simulink subsystem "KF_prediction"  (R2021a)
settings: Solver=VariableStepAuto  StartTime=0.0  StopTime=10.0  RelTol=1e-3
undefined symbols (not defined in the file): gyro_bias_init, gyro_std, magnitude
libraries: dspmtrx3 x5
settings Model: Creator=Laura  LastModifiedBy=Laura

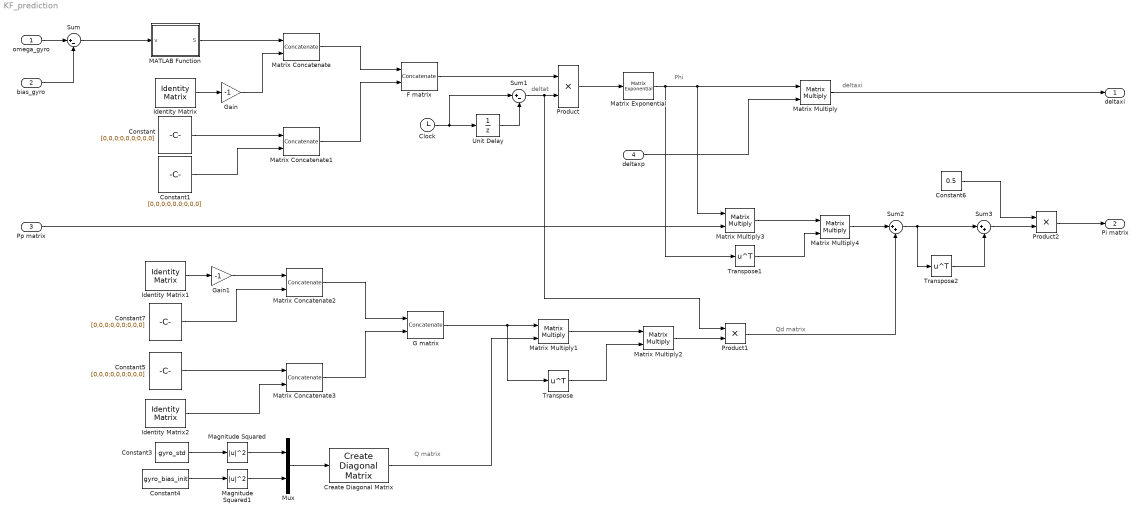
== system KF_prediction ==
  note: Qd matrix
  note: Q matrix
  note: Phi
  note: deltaxi
  note: deltat
  omega_gyro : Inport
  bias_gyro : Inport  Port=2
  Pp matrix : Inport  Port=3
  deltaxp : Inport  Port=4
  Clock : Clock
  Constant{,1,5,7} (4 alike) : Constant  Value=[0,0,0;0,0,0;0,0,0]
  Constant3 : Constant  Value=gyro_std
  Constant4 : Constant  Value=gyro_bias_init
  Constant6 : Constant  Value=0.5
  Create Diagonal Matrix : dspmtrx3/Create Diagonal Matrix
      settings: SourceProductBaseCode=DS
  F matrix : Concatenate  Mode=Multidimensional array
  G matrix : Concatenate  Mode=Multidimensional array
  Gain : Gain  Gain=-1
  Gain1 : Gain  Gain=-1
  Identity Matrix : dspmtrx3/Identity Matrix  Inherit=off  N=3  Ts=1  dataType=double  isSigned=on  wordLen=16  udDataType=sfix(16)  fracBitsMode=Best precision  numFracBits=15  OutDataTypeStr=double  LastOutDataTypeStr=double
  Identity Matrix1 : dspmtrx3/Identity Matrix  Inherit=off  N=3  Ts=1  dataType=double  isSigned=on  wordLen=16  udDataType=sfix(16)  fracBitsMode=Best precision  numFracBits=15  OutDataTypeStr=double  LastOutDataTypeStr=double
  Identity Matrix2 : dspmtrx3/Identity Matrix  Inherit=off  N=3  Ts=1  dataType=double  isSigned=on  wordLen=16  udDataType=sfix(16)  fracBitsMode=Best precision  numFracBits=15  OutDataTypeStr=double  LastOutDataTypeStr=double
  MATLAB Function : MATLAB Function  TreatAsAtomicUnit=on
  Magnitude Squared : Math  Operator=magnitude^2  SaturateOnIntegerOverflow=on
  Magnitude Squared1 : Math  Operator=magnitude^2  SaturateOnIntegerOverflow=on
  Matrix Concatenate{,1..3} (4 alike) : Concatenate  Mode=Multidimensional array  ConcatenateDimension=2
  Matrix Exponential : dspmtrx3/Matrix Exponential
      settings: SourceProductBaseCode=DS
  Matrix Multiply{,1..4} (5 alike) : Product  Multiplication=Matrix(*)
  Mux : Mux  Inputs=2
  Product : Product
  Product1 : Product
  Product2 : Product
  Sum : Sum  Inputs=|+-
  Sum1 : Sum  Inputs=|+-
  Sum2 : Sum  Inputs=|++
  Sum3 : Sum  Inputs=|++
  Transpose : Math  Operator=transpose  SaturateOnIntegerOverflow=on
  Transpose1 : Math  Operator=transpose  SaturateOnIntegerOverflow=on
  Transpose2 : Math  Operator=transpose  SaturateOnIntegerOverflow=on
  Unit Delay : UnitDelay  SampleTime=-1  HasFrameUpgradeWarning=on
  deltaxi : Outport
  Pi matrix : Outport  Port=2
  wires:
  omega_gyro/1 -> Sum/1
  Sum/1 -> MATLAB Function/1(v)
  Identity Matrix/1 -> Gain/1
  Gain/1 -> Matrix Concatenate/2
  MATLAB Function/1(S) -> Matrix Concatenate/1
  Constant/1 -> Matrix Concatenate1/1
  Constant1/1 -> Matrix Concatenate1/2
  Matrix Concatenate/1 -> F matrix/1
  Matrix Concatenate1/1 -> F matrix/2
  Clock/1 -> Sum1/1, Unit Delay/1
  F matrix/1 -> Product/1
  Product/1 -> Matrix Exponential/1
  Sum1/1 -> Product1/1, Product/2
  Matrix Exponential/1 -> Transpose1/1, Matrix Multiply3/1, Matrix Multiply/1
  Matrix Multiply/1 -> deltaxi/1
  Constant5/1 -> Matrix Concatenate3/1
  Identity Matrix1/1 -> Gain1/1
  Gain1/1 -> Matrix Concatenate2/1
  Constant7/1 -> Matrix Concatenate2/2
  Identity Matrix2/1 -> Matrix Concatenate3/2
  Matrix Concatenate2/1 -> G matrix/1
  Matrix Concatenate3/1 -> G matrix/2
  Constant4/1 -> Magnitude Squared1/1
  Magnitude Squared1/1 -> Mux/2
  Magnitude Squared/1 -> Mux/1
  Mux/1 -> Create Diagonal Matrix/1
  Constant3/1 -> Magnitude Squared/1
  G matrix/1 -> Transpose/1, Matrix Multiply1/1
  Create Diagonal Matrix/1 -> Matrix Multiply1/2
  Transpose/1 -> Matrix Multiply2/2
  Matrix Multiply1/1 -> Matrix Multiply2/1
  Unit Delay/1 -> Sum1/2
  Matrix Multiply2/1 -> Product1/2
  bias_gyro/1 -> Sum/2
  Pp matrix/1 -> Matrix Multiply3/2
  Matrix Multiply3/1 -> Matrix Multiply4/1
  Transpose1/1 -> Matrix Multiply4/2
  Matrix Multiply4/1 -> Sum2/1
  Product1/1 -> Sum2/2
  Sum2/1 -> Transpose2/1, Sum3/1
  Transpose2/1 -> Sum3/2
  Sum3/1 -> Product2/2
  Constant6/1 -> Product2/1
  Product2/1 -> Pi matrix/1
  deltaxp/1 -> Matrix Multiply/2

== matlab function KF_prediction/MATLAB Function ==
  data: v input; S output
function S = skewm(v)
% skewm forms a skew-symmetric matrix from a 3x1 vector
%
% INPUT
%              v, 3x1 vector
%
%	OUTPUT
%              S, 3x3 skew-symmetric matrix
%
%%
    x = v(1);
    y = v(2);
    z = v(3);

    S = [ 0 -z   y;
          z  0  -x;
         -y  x   0];

end
